simulink model "CarritoDiferencial"  (R2015a)
settings: Solver=ode4  StartTime=0.0  StopTime=50  FixedStep=.01  RelTol=1e-3
libraries: simulink x2
settings Model: Creator=Sala6  LastModifiedBy=Sala6

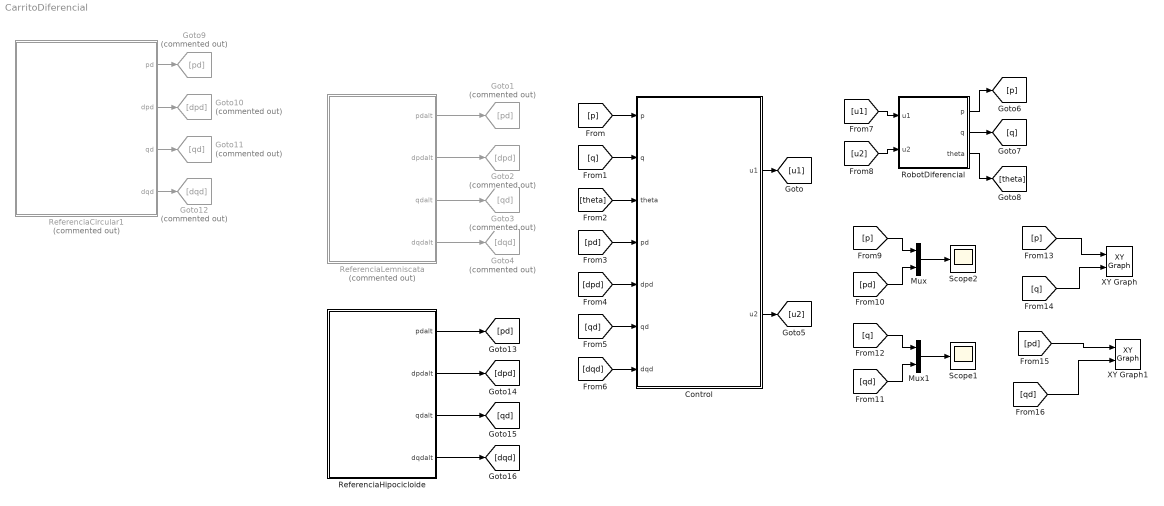
== system CarritoDiferencial ==
  Control : Subsystem  mask{kpp=200, kpq=200, rho=.1}
      mask prompts: kpp "Constante proporcional (kpp)"; kpq "Constante proporcional (kpq)"; rho "Excentricidad(rho)"
  Goto1 : Goto  Commented=on  GotoTag=pd
  Goto10 : Goto  Commented=on  GotoTag=dpd
  Goto11 : Goto  Commented=on  GotoTag=qd
  Goto12 : Goto  Commented=on  GotoTag=dqd
  Goto2 : Goto  Commented=on  GotoTag=dpd
  Goto3 : Goto  Commented=on  GotoTag=qd
  Goto4 : Goto  Commented=on  GotoTag=dqd
  Goto9 : Goto  Commented=on  GotoTag=pd
  Mux : Mux  Inputs=2
  Mux1 : Mux  Inputs=2
  ReferenciaCircular1 : Subsystem  Commented=on  mask{A=.5, w=pi/20}
      mask prompts: A "Radio"; w "Frecuencia"
  ReferenciaHipocicloide : Subsystem  mask{r=.5, k=10}
  ReferenciaLemniscata : Subsystem  Commented=on  mask{A=.5, w=pi/20}
      mask prompts: A "Radio"; w "Frecuencia"
  RobotDiferencial : Subsystem  mask{p0=-3, q0=-3, theta0=0, rho=.1}
      mask prompts: p0 "Posicion inicial(p0)"; q0 "Posicion inicial(q0)"; theta0 "Orientacion inicial(theta0)"; rho "Excentricidad(rho)"
  Scope1 : Scope
  Scope2 : Scope
      settings: YMin=-12  YMax=12
  XY Graph : simulink/Sinks/XY Graph  xmin=-10  xmax=10  ymin=-10  ymax=10  st=-1
  XY Graph1 : simulink/Sinks/XY Graph  xmin=-10  xmax=10  ymin=-10  ymax=10  st=-1
  wires:
  [p] -> Control/1("p ")
  [q] -> Control/2(q)
  [theta] -> Control/3(theta)
  [pd] -> Control/4(pd)
  [dpd] -> Control/5(dpd)
  [qd] -> Control/6(qd)
  [dqd] -> Control/7(dqd)
  Control/1(u1) -> [u1]
  Control/2(u2) -> [u2]
  [u1] -> RobotDiferencial/1("u1 ")
  [u2] -> RobotDiferencial/2(u2)
  RobotDiferencial/1(p) -> [p]
  RobotDiferencial/2(q) -> [q]
  RobotDiferencial/3(theta) -> [theta]
  Mux/1 -> Scope2/1
  [pd] -> Mux/2
  [p] -> Mux/1
  Mux1/1 -> Scope1/1
  [qd] -> Mux1/2
  [q] -> Mux1/1
  ReferenciaLemniscata/1(pdalt) -> Goto1/1
  ReferenciaLemniscata/2(dpdalt) -> Goto2/1
  ReferenciaLemniscata/3(qdalt) -> Goto3/1
  ReferenciaLemniscata/4(dqdalt) -> Goto4/1
  ReferenciaCircular1/1(pd) -> Goto9/1
  ReferenciaCircular1/2(dpd) -> Goto10/1
  ReferenciaCircular1/3(qd) -> Goto11/1
  ReferenciaCircular1/4("dqd ") -> Goto12/1
  ReferenciaHipocicloide/1(pdalt) -> [pd]
  ReferenciaHipocicloide/2(dpdalt) -> [dpd]
  ReferenciaHipocicloide/4(dqdalt) -> [dqd]
  ReferenciaHipocicloide/3(qdalt) -> [qd]
  [p] -> XY Graph/1
  [q] -> XY Graph/2
  [pd] -> XY Graph1/1
  [qd] -> XY Graph1/2

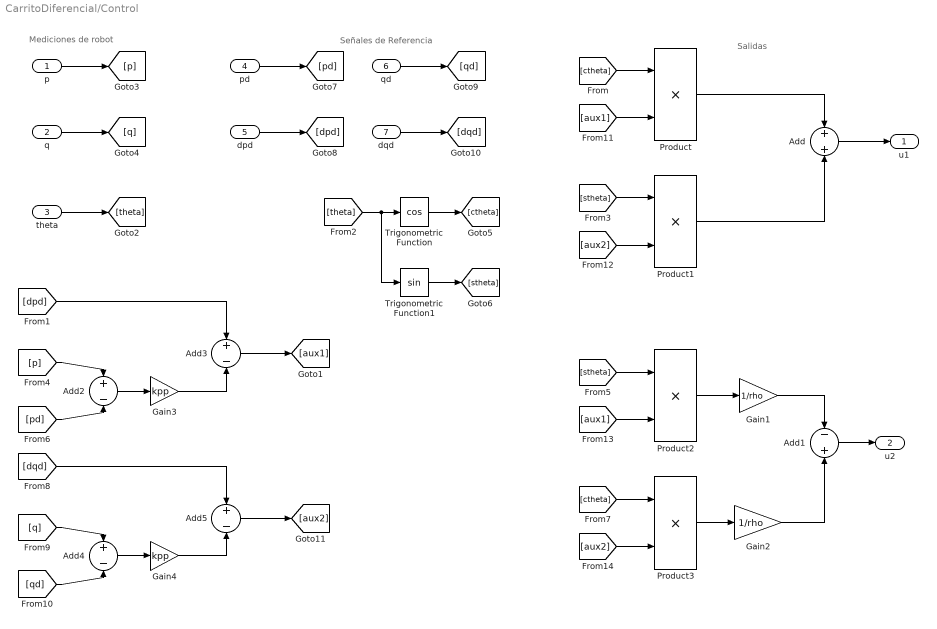
== system CarritoDiferencial/Control ==
  note: Salidas
  note: Mediciones de robot
  note: Señales de Referencia
  "p " : Inport
  q : Inport  Port=2
  theta : Inport  Port=3
  pd : Inport  Port=4
  dpd : Inport  Port=5
  qd : Inport  Port=6
  dqd : Inport  Port=7
  Add : Sum
  Add1 : Sum  Inputs=-+
  Add{2..5} (4 alike) : Sum  Inputs=+-
  Gain1 : Gain  Gain=1/rho
  Gain2 : Gain  Gain=1/rho
  Gain3 : Gain  Gain=kpp
  Gain4 : Gain  Gain=kpp
  Product{,1..3} (4 alike) : Product
  Trigonometric Function : Trigonometry  Operator=cos
  Trigonometric Function1 : Trigonometry
  u1 : Outport
  u2 : Outport  Port=2
  wires:
  Gain2/1 -> Add1/2
  [stheta] -> Product2/1
  Product2/1 -> Gain1/1
  [ctheta] -> Product3/1
  Product3/1 -> Gain2/1
  Trigonometric Function/1 -> [ctheta]
  Product1/1 -> Add/2
  Product/1 -> Add/1
  q/1 -> [q]
  [stheta] -> Product1/1
  Trigonometric Function1/1 -> [stheta]
  [theta] -> Trigonometric Function/1, Trigonometric Function1/1
  "p "/1 -> [p]
  [ctheta] -> Product/1
  theta/1 -> [theta]
  pd/1 -> [pd]
  dpd/1 -> [dpd]
  qd/1 -> [qd]
  dqd/1 -> [dqd]
  [p] -> Add2/1
  [pd] -> Add2/2
  Add2/1 -> Gain3/1
  [dpd] -> Add3/1
  Gain3/1 -> Add3/2
  Add3/1 -> [aux1]
  [q] -> Add4/1
  [qd] -> Add4/2
  Add4/1 -> Gain4/1
  [dqd] -> Add5/1
  Gain4/1 -> Add5/2
  Add5/1 -> [aux2]
  [aux1] -> Product/2
  [aux2] -> Product1/2
  Add/1 -> u1/1
  Add1/1 -> u2/1
  Gain1/1 -> Add1/1
  [aux1] -> Product2/2
  [aux2] -> Product3/2

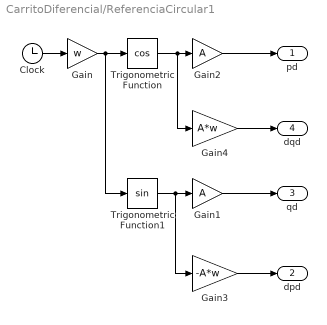
== system CarritoDiferencial/ReferenciaCircular1 ==
  Clock : Clock
  Gain : Gain  Gain=w
  Gain1 : Gain  Gain=A
  Gain2 : Gain  Gain=A
  Gain3 : Gain  Gain=-A*w
  Gain4 : Gain  Gain=A*w
  Trigonometric Function : Trigonometry  Operator=cos
  Trigonometric Function1 : Trigonometry
  pd : Outport
  dpd : Outport  Port=2
  qd : Outport  Port=3
  "dqd " : Outport  Port=4
  wires:
  Gain4/1 -> "dqd "/1
  Gain3/1 -> dpd/1
  Trigonometric Function/1 -> Gain2/1, Gain4/1
  Gain/1 -> Trigonometric Function/1, Trigonometric Function1/1
  Gain1/1 -> qd/1
  Trigonometric Function1/1 -> Gain1/1, Gain3/1
  Clock/1 -> Gain/1
  Gain2/1 -> pd/1

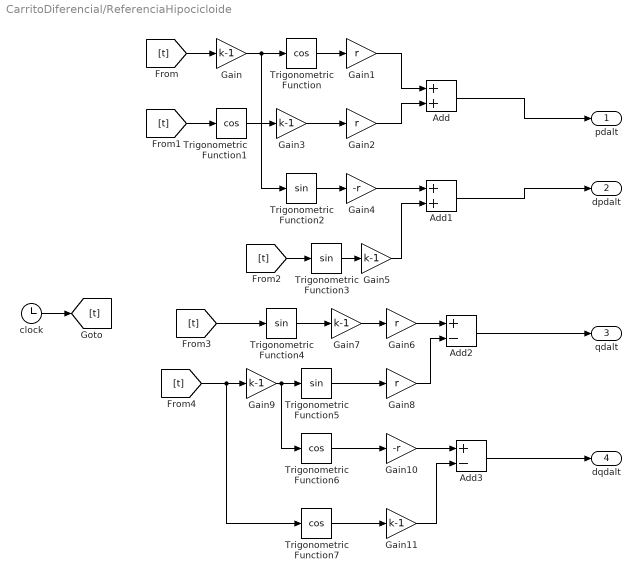
== system CarritoDiferencial/ReferenciaHipocicloide ==
  Add : Sum
  Add1 : Sum
  Add2 : Sum  Inputs=+-
  Add3 : Sum  Inputs=+-
  Gain{,3,5,7,9,11} (6 alike) : Gain  Gain=k-1
  Gain{1..2,6,8} (4 alike) : Gain  Gain=r
  Gain10 : Gain  Gain=-r
  Gain4 : Gain  Gain=-r
  Trigonometric Function{,1,6..7} (4 alike) : Trigonometry  Operator=cos
  Trigonometric Function{2..5} (4 alike) : Trigonometry
  clock : Clock
  pdalt : Outport
  dpdalt : Outport  Port=2
  qdalt : Outport  Port=3
  dqdalt : Outport  Port=4
  wires:
  clock/1 -> [t]
  [t] -> Gain/1
  Gain/1 -> Trigonometric Function2/1, Trigonometric Function/1
  Trigonometric Function/1 -> Gain1/1
  Gain1/1 -> Add/1
  Trigonometric Function1/1 -> Gain3/1
  Gain2/1 -> Add/2
  [t] -> Trigonometric Function1/1
  Gain3/1 -> Gain2/1
  Add/1 -> pdalt/1
  Trigonometric Function2/1 -> Gain4/1
  Gain4/1 -> Add1/1
  Trigonometric Function3/1 -> Gain5/1
  [t] -> Trigonometric Function3/1
  Gain5/1 -> Add1/2
  Add1/1 -> dpdalt/1
  [t] -> Trigonometric Function4/1
  Gain7/1 -> Gain6/1
  Trigonometric Function4/1 -> Gain7/1
  Gain6/1 -> Add2/1
  Trigonometric Function5/1 -> Gain8/1
  [t] -> Trigonometric Function7/1, Gain9/1
  Gain8/1 -> Add2/2
  Add2/1 -> qdalt/1
  Trigonometric Function6/1 -> Gain10/1
  Gain9/1 -> Trigonometric Function6/1, Trigonometric Function5/1
  Gain10/1 -> Add3/1
  Add3/1 -> dqdalt/1
  Trigonometric Function7/1 -> Gain11/1
  Gain11/1 -> Add3/2

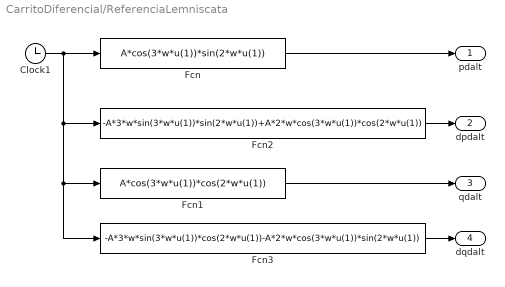
== system CarritoDiferencial/ReferenciaLemniscata ==
  Clock1 : Clock
  Fcn : Fcn  Expr=A*cos(3*w*u(1))*sin(2*w*u(1))
  Fcn1 : Fcn  Expr=A*cos(3*w*u(1))*cos(2*w*u(1))
  Fcn2 : Fcn  Expr=-A*3*w*sin(3*w*u(1))*sin(2*w*u(1))+A*2*w*cos(3*w*u(1))*cos(2*w*u(1))
  Fcn3 : Fcn  Expr=-A*3*w*sin(3*w*u(1))*cos(2*w*u(1))-A*2*w*cos(3*w*u(1))*sin(2*w*u(1))
  pdalt : Outport
  dpdalt : Outport  Port=2
  qdalt : Outport  Port=3
  dqdalt : Outport  Port=4
  wires:
  Clock1/1 -> Fcn2/1, Fcn1/1, Fcn3/1, Fcn/1
  Fcn/1 -> pdalt/1
  Fcn2/1 -> dpdalt/1
  Fcn1/1 -> qdalt/1
  Fcn3/1 -> dqdalt/1

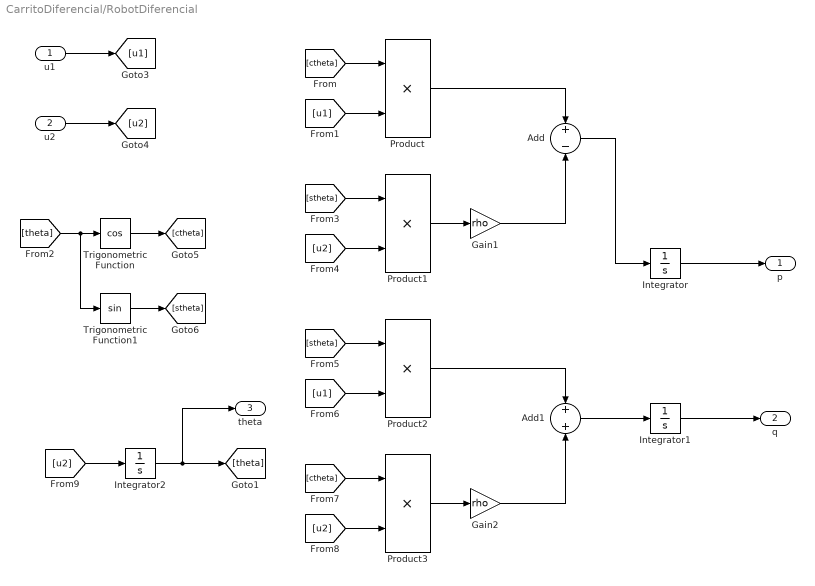
== system CarritoDiferencial/RobotDiferencial ==
  "u1 " : Inport
  u2 : Inport  Port=2
  Add : Sum  Inputs=+-
  Add1 : Sum
  Gain1 : Gain  Gain=rho
  Gain2 : Gain  Gain=rho
  Integrator : Integrator  InitialCondition=p0
  Integrator1 : Integrator  InitialCondition=q0
  Integrator2 : Integrator  InitialCondition=theta0
  Product{,1..3} (4 alike) : Product
  Trigonometric Function : Trigonometry  Operator=cos
  Trigonometric Function1 : Trigonometry
  p : Outport
  q : Outport  Port=2
  theta : Outport  Port=3
  wires:
  Integrator/1 -> p/1
  [ctheta] -> Product/1
  Integrator2/1 -> theta/1, [theta]
  Integrator1/1 -> q/1
  "u1 "/1 -> [u1]
  [theta] -> Trigonometric Function1/1, Trigonometric Function/1
  Trigonometric Function1/1 -> [stheta]
  Product1/1 -> Gain1/1
  [u2] -> Product1/2
  Add/1 -> Integrator/1
  [stheta] -> Product1/1
  [u1] -> Product/2
  u2/1 -> [u2]
  Product/1 -> Add/1
  Gain1/1 -> Add/2
  Trigonometric Function/1 -> [ctheta]
  Product3/1 -> Gain2/1
  [u2] -> Product3/2
  [u1] -> Product2/2
  [ctheta] -> Product3/1
  Product2/1 -> Add1/1
  [stheta] -> Product2/1
  Gain2/1 -> Add1/2
  [u2] -> Integrator2/1
  Add1/1 -> Integrator1/1
